simulink model "traj_ref"  (R2020b)
settings: Solver=VariableStepAuto  StartTime=0.0  StopTime=500  RelTol=1e-3
libraries: simulink x7, shared3dof x1, pid_lib x1
settings Model: Creator=Hariharan  LastModifiedBy=Hariharan

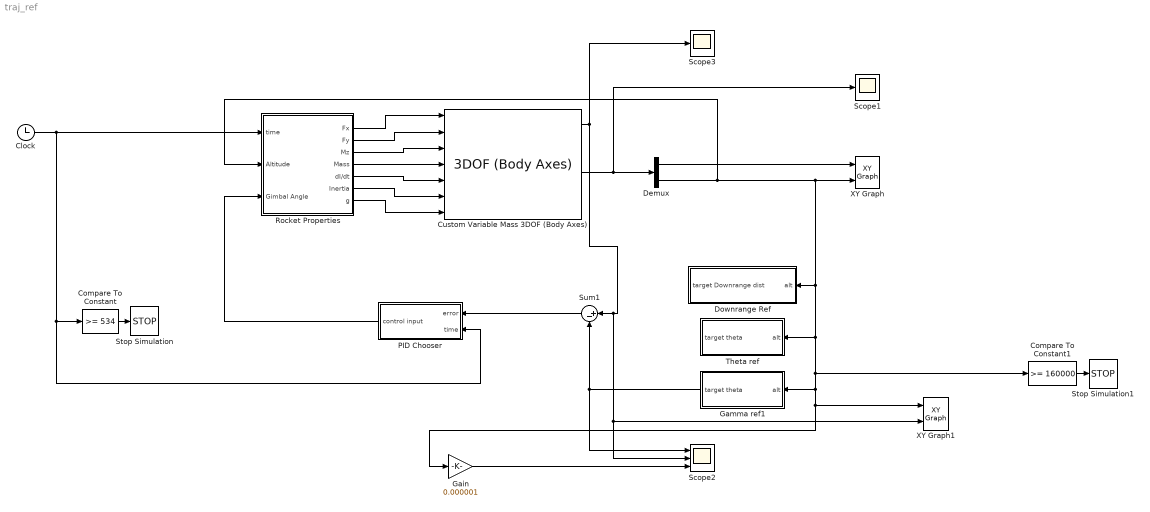
== system traj_ref ==
  Clock : Clock
  Compare To Constant : simulink/Logic and Bit Operations/Compare To Constant  relop=>=  const=534  OutDataTypeStr=boolean
  Compare To Constant1 : simulink/Logic and Bit Operations/Compare To Constant  relop=>=  const=160000  OutDataTypeStr=boolean
  Custom Variable Mass 3DOF (Body Axes) : shared3dof/3DOF (Body Axes)  units=Metric (MKS)  mtype=Custom Variable  v_ini=0  theta_ini=1.57  alpha_ini=0  pos_ini=[0 0]  q_ini=0  mass=1.0  mass_e=0.5  mass_f=3.0  Iyy=1.0  Iyy_e=0.5  Iyy_f=3.0  g_in=External  g=9.81  vre_flag=off  abi_flag=off  aMode=0  vel_statename=''  theta_statename=''  pos_statename=''  q_statename=''  mass_statename=''
      settings: SourceProductBaseCode=AE,PW,MT,UV,VE,VP
  Demux : Demux  Outputs=2
  Downrange Ref : Subsystem
  Gain : Gain  Gain=0.000001
  Gamma ref1 : Subsystem
  PID Chooser : Subsystem
  Rocket Properties : Subsystem
  Scope1 : Scope
  Scope2 : Scope  NumInputPorts=3
  Scope3 : Scope
  Stop Simulation : Stop
  Stop Simulation1 : Stop
  Sum1 : Sum  Inputs=|+-
  Theta ref : Subsystem
  XY Graph : simulink/Sinks/XY Graph  xmin=0  xmax=60000  ymin=0  ymax=450000  st=1
  XY Graph1 : simulink/Sinks/XY Graph  xmin=0  xmax=150000  ymin=-0.2  ymax=1.6  st=1
  wires:
  Rocket Properties/1(Fx) -> Custom Variable Mass 3DOF (Body Axes)/1
  Rocket Properties/2(Fy) -> Custom Variable Mass 3DOF (Body Axes)/2
  Rocket Properties/3(Mz) -> Custom Variable Mass 3DOF (Body Axes)/3
  Rocket Properties/4(Mass) -> Custom Variable Mass 3DOF (Body Axes)/4
  Rocket Properties/5(dI/dt) -> Custom Variable Mass 3DOF (Body Axes)/5
  Rocket Properties/6(Inertia) -> Custom Variable Mass 3DOF (Body Axes)/6
  Clock/1 -> Rocket Properties/1(time), PID Chooser/2(time), Compare To Constant/1
  Custom Variable Mass 3DOF (Body Axes)/4 -> Scope1/1, Demux/1
  Demux/1 -> XY Graph/1
  Compare To Constant/1 -> Stop Simulation/1
  Rocket Properties/7(g) -> Custom Variable Mass 3DOF (Body Axes)/7
  Sum1/1 -> PID Chooser/1(error)
  PID Chooser/1(control input) -> Rocket Properties/3(Gimbal Angle)
  Gamma ref1/1(target theta) -> Scope2/1, Sum1/2
  Gain/1 -> Scope2/3
  Demux/2 -> Rocket Properties/2(Altitude), XY Graph/2, Downrange Ref/1(alt), XY Graph1/1, Gain/1, Gamma ref1/1(alt), Compare To Constant1/1, Theta ref/1(alt)
  Custom Variable Mass 3DOF (Body Axes)/1 -> Scope3/1, Scope2/2, XY Graph1/2, Sum1/1
  Compare To Constant1/1 -> Stop Simulation1/1

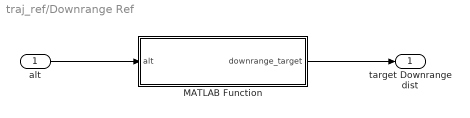
== system traj_ref/Downrange Ref ==
  alt : Inport
  MATLAB Function : MATLAB Function  TreatAsAtomicUnit=on
  target Downrange dist : Outport
  wires:
  alt/1 -> MATLAB Function/1(alt)
  MATLAB Function/1(downrange_target) -> target Downrange dist/1

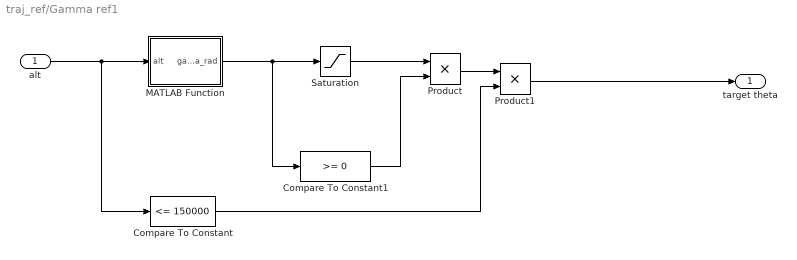
== system traj_ref/Gamma ref1 ==
  alt : Inport
  Compare To Constant : simulink/Logic and Bit Operations/Compare To Constant  relop=<=  const=150000  OutDataTypeStr=boolean
  Compare To Constant1 : simulink/Logic and Bit Operations/Compare To Constant  relop=>=  const=0  OutDataTypeStr=boolean
  MATLAB Function : MATLAB Function  TreatAsAtomicUnit=on
  Product : Product
  Product1 : Product
  Saturation : Saturate  UpperLimit=1.58  LowerLimit=-0.2
  target theta : Outport
  wires:
  MATLAB Function/1(gamma_rad) -> Compare To Constant1/1, Saturation/1
  Saturation/1 -> Product/1
  alt/1 -> Compare To Constant/1, MATLAB Function/1(alt)
  Compare To Constant1/1 -> Product/2
  Product/1 -> Product1/1
  Product1/1 -> target theta/1
  Compare To Constant/1 -> Product1/2

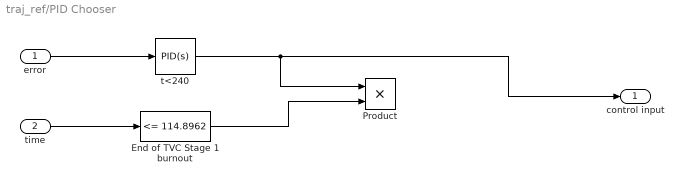
== system traj_ref/PID Chooser ==
  error : Inport
  time : Inport  Port=2
  End of TVC Stage 1 burnout : simulink/Logic and Bit Operations/Compare To Constant  relop=<=  const=114.8962  OutDataTypeStr=boolean
  Product : Product
  t<240 : pid_lib/PID Controller  Controller=PID  Form=Parallel  TimeDomain=Continuous-time  UseExternalTs=off  SampleTime=-1  IntegratorMethod=Forward Euler  FilterMethod=Forward Euler  ControllerParametersSource=internal  P=-0.326668319119736  I=-0.193796986247956  D=-0.10856262264642  UseFilter=on  N=23.7880653667222  TunerSelectOption=Transfer Function Based (PID Tuner App)  InitialConditionSource=internal  InitialConditionForIntegrator=0  InitialConditionForFilter=0  DifferentiatorICPrevScaledInput=0  ExternalReset=none  TrackingMode=off  Kt=1  LimitOutput=off  SatLimitsSource=internal  UpperSaturationLimit=inf  LowerSaturationLimit=-inf  LinearizeAsGain=on  AntiWindupMode=none  Kb=1  POutMin=[]  POutMax=[]  IOutMin=[]  IOutMax=[]  DOutMin=[]  DOutMax=[]  NOutMin=[]  NOutMax=[]  SumOutMin=[]  SumOutMax=[]  SaturationOutMin=[]  SaturationOutMax=[]  PParamMin=[]  PParamMax=[]  IParamMin=[]  IParamMax=[]  DParamMin=[]  DParamMax=[]  NParamMin=[]  NParamMax=[]  KbParamMin=[]  KbParamMax=[]  KtParamMin=[]  KtParamMax=[]  KbOutMin=[]  KbOutMax=[]  KtOutMin=[]  KtOutMax=[]  IntegratorOutMin=[]  IntegratorOutMax=[]  FilterOutMin=[]  FilterOutMax=[]  SumI1OutMin=[]  SumI1OutMax=[]  SumI2OutMin=[]  SumI2OutMax=[]  SumI3OutMin=[]  SumI3OutMax=[]  SumI4OutMin=[]  SumI4OutMax=[]  SumDOutMin=[]  SumDOutMax=[]  DifferentiatorOutMin=[]  DifferentiatorOutMax=[]  FilterDiffOutCoefMin=[]  FilterDiffOutCoefMax=[]  ReciprocalOutMin=[]  ReciprocalOutMax=[]  SumDenOutMin=[]  SumDenOutMax=[]  SumNumOutMin=[]  SumNumOutMax=[]  DivideOutMin=[]  DivideOutMax=[]  UdiffTsProdOutMin=[]  UdiffTsProdOutMax=[]  NTsProdOutMin=[]  NTsProdOutMax=[]  UintegralTsProdOutMin=[]  UintegralTsProdOutMax=[]  UngainTsProdOutMin=[]  UngainTsProdOutMax=[]  IntegratorContinuousStateAttributes=''  IntegratorStateMustResolveToSignalObject=off  IntegratorRTWStateStorageClass=Auto  FilterContinuousStateAttributes=''  FilterStateMustResolveToSignalObject=off  FilterRTWStateStorageClass=Auto  ParallelPVariant=InternalParameters  IdealPVariant=Disabled  IVariant=InternalParameters  DVariant=InternalParameters  IntegratorVariant=Continuous  SatVariant=Disabled  AWVariant=Passthrough  PCopyVariant=Disabled  TRVariant=Disabled  FdbkBlocksVariant=Forward  IdealPFdbkVariant=Disabled  SatFdbkVariant=Disabled  DerivativeFilterVariant=ContFilter  NVariant=InternalParameters  NCopyVariant=Disabled  FilterICVariant=InternalICsFilter  IntegratorICVariant=InternalICs  ExternalResetVariant=Disabled  TRSumVariant=Passthrough  SumFdbkVariant=Disabled  SumVariant=Sum_PID  TsampFilterVariant=InternalTs  TsampNgainVariant=Passthrough  TsampIntegralVariant=Passthrough  ExternalSaturationOutDataTypeStr=Inherit: Same as second input
  control input : Outport
  wires:
  time/1 -> End of TVC Stage 1 burnout/1
  error/1 -> t<240/1
  End of TVC Stage 1 burnout/1 -> Product/2
  t<240/1 -> control input/1, Product/1

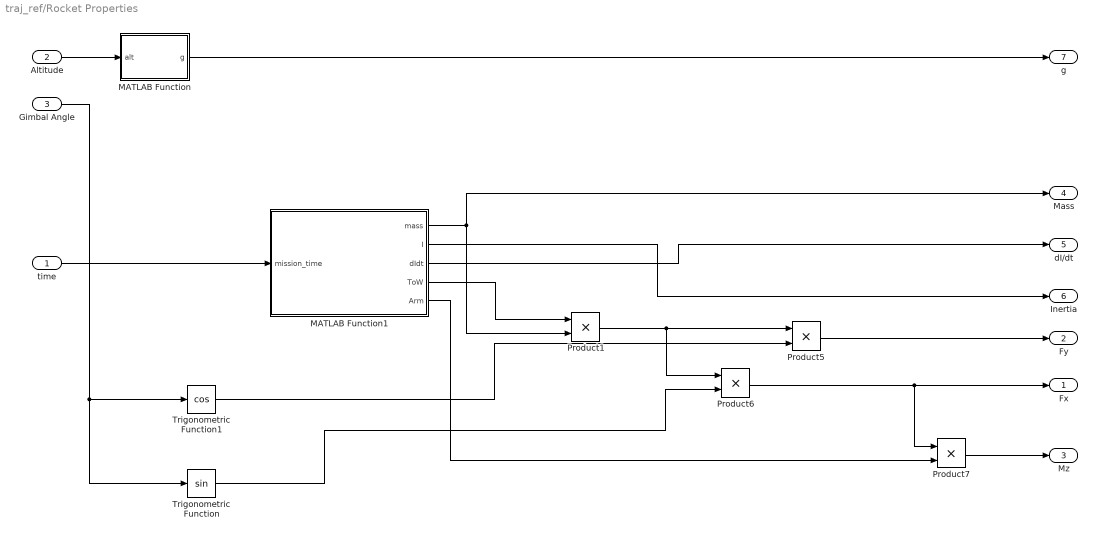
== system traj_ref/Rocket Properties ==
  time : Inport
  Altitude : Inport  Port=2
  Gimbal Angle : Inport  Port=3
  MATLAB Function : MATLAB Function  TreatAsAtomicUnit=on
  MATLAB Function1 : MATLAB Function  TreatAsAtomicUnit=on
  Product{1,5..7} (4 alike) : Product
  Trigonometric Function : Trigonometry
  Trigonometric Function1 : Trigonometry  Operator=cos
  Fx : Outport
  Fy : Outport  Port=2
  Mz : Outport  Port=3
  Mass : Outport  Port=4
  dI/dt : Outport  Port=5
  Inertia : Outport  Port=6
  g : Outport  Port=7
  wires:
  Altitude/1 -> MATLAB Function/1(alt)
  time/1 -> MATLAB Function1/1(mission_time)
  MATLAB Function1/3(dIdt) -> dI/dt/1
  MATLAB Function1/2(I) -> Inertia/1
  MATLAB Function1/5(Arm) -> Product7/2
  MATLAB Function1/4(ToW) -> Product1/1
  Gimbal Angle/1 -> Trigonometric Function/1, Trigonometric Function1/1
  MATLAB Function/1(g) -> g/1
  MATLAB Function1/1(mass) -> Product1/2, Mass/1
  Product1/1 -> Product6/1, Product5/1
  Trigonometric Function1/1 -> Product5/2
  Trigonometric Function/1 -> Product6/2
  Product5/1 -> Fy/1
  Product6/1 -> Product7/1, Fx/1
  Product7/1 -> Mz/1

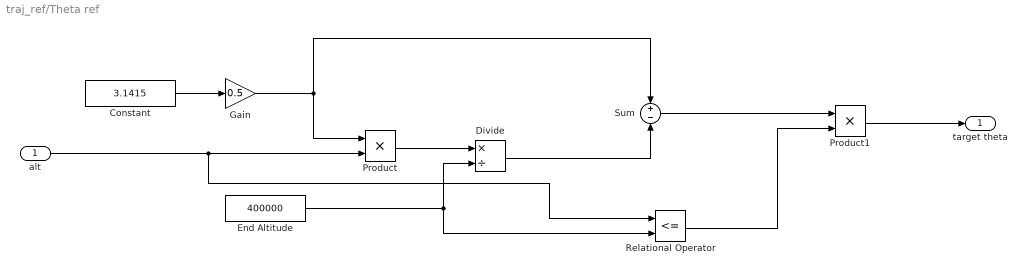
== system traj_ref/Theta ref ==
  alt : Inport
  Constant : Constant  Value=3.1415
  Divide : Product  Inputs=*/
  End Altitude : Constant  Value=400000
  Gain : Gain  Gain=0.5
  Product : Product
  Product1 : Product
  Relational Operator : RelationalOperator  Operator=<=  OutDataTypeStr=boolean  RndMeth=Simplest
  Sum : Sum  Inputs=+-
  target theta : Outport
  wires:
  Product/1 -> Divide/1
  Constant/1 -> Gain/1
  End Altitude/1 -> Relational Operator/2, Divide/2
  Gain/1 -> Sum/1, Product/1
  Divide/1 -> Sum/2
  alt/1 -> Relational Operator/1, Product/2
  Sum/1 -> Product1/1
  Relational Operator/1 -> Product1/2
  Product1/1 -> target theta/1

== matlab function traj_ref/Rocket Properties/MATLAB Function1 ==
  data: mission_time input; mass output; I output; dIdt output; ToW output; Arm output
function [mass,I,dIdt,ToW,Arm] = rocket_prop_eval(mission_time)

L = [14.52 1.95 1.83];

tbb = [114.8962  156.7683  261.4940];

m0 = [1.1112e4    0.1664e4    0.0239e4];

M0 = 1.3065e+04;

m_dot = [69.2893    7.4443    0.5640];

Diam = 0.83;

thick = 0.001;


if mission_time < tbb(1)
        
        m_dot_current = m_dot(1);
        
        mass = M0 - (m_dot(1)*mission_time);
        
        Length = sum(L);
        
        ToW = 2;
        
    elseif (mission_time >= tbb(1)) && (mission_time < sum(tbb(1:2)))
        
        m_dot_current = m_dot(2);
        
        mass = M0 - m0(1) - (m_dot(2)*(mission_time - tbb(1))); 
        
        Length = sum(L(2:end));
        
        ToW = 2;
        
    else
        
        m_dot_current = m_dot(3);
        
        mass = M0 - m0(1) - m0(2) - (m_dot(3)*(mission_time - tbb(1) - tbb(2)));
        
        Length = sum(L(end));
        
        ToW = 1000/mass;
        
end
    
I = 0.5*mass*(Diam/2)^2;

dIdt = m_dot_current;

Arm = Length/2;

end

== matlab function traj_ref/Rocket Properties/MATLAB Function ==
  data: alt input; g output
function g = g_calc(alt)

Mu = 3.986004418e14;
Re = 6.371e6;

R = Re + alt;

g = (Mu/(R^2));

end

== matlab function traj_ref/Downrange Ref/MATLAB Function ==
  data: alt input; downrange_target output
function downrange_target = traj_ref(alt)

downrange_target = -5e-32*(alt^6) + 4e-25*(alt^5) - 1e-18*(alt^4) + 2e-12*(alt^3) - 1e-06*(alt^2) + 0.5577*(alt) + 2793.1;

end

== matlab function traj_ref/Gamma ref1/MATLAB Function ==
  data: alt input; gamma_rad output
function gamma_rad = target_gamma(alt)

%gamma_rad = 4e-30*(alt)^6 - 2e-24*(alt)^5 + 4e-19*(alt)^4 - 4e-14*(alt)^3 + 3e-09*(alt)^2 - 8e-05*(alt) + 1.399;

x = alt;

   p1 =   1.561e-39;  %(1.485e-39, 1.637e-39)
   p2 =  -1.005e-33;  %(-1.05e-33, -9.592e-34)
   p3 =   2.688e-28;  %(2.576e-28, 2.801e-28)
   p4 =  -3.881e-23;  %(-4.028e-23, -3.734e-23)
   p5 =   3.296e-18;  %(3.187e-18, 3.405e-18)
   p6 =  -1.701e-13;  %(-1.746e-13, -1.655e-13)
   p7 =   5.433e-09;  %(5.332e-09, 5.534e-09)
   p8 =  -0.0001119;  %(-0.0001129, -0.0001109)
   p9 =       1.464;  %(1.46, 1.467)
       
  gamma_rad = p1*x^8 + p2*x^7 + p3*x^6 + p4*x^5 + p5*x^4 + p6*x^3 + p7*x^2 + p8*x + p9;

end
